simulink model "Model_8"  (R2020b)
settings: Solver=VariableStepAuto  StartTime=0.0  StopTime=10.0  RelTol=1e-3
settings Model: Creator=samar  LastModifiedBy=samar

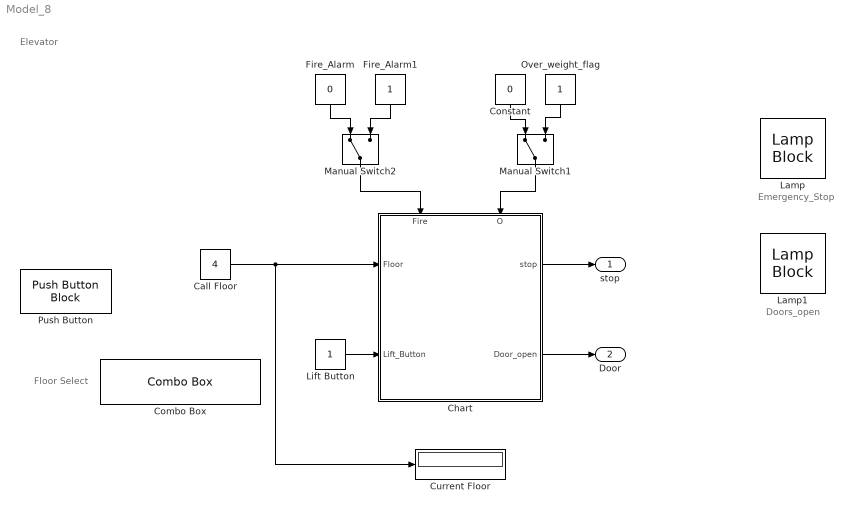
== system Model_8 ==
  note: Doors_open
  note: Emergency_Stop
  note: Floor Select
  note: Elevator
  Call Floor : Constant  Value=4
  Chart : Stateflow chart  TreatAsAtomicUnit=on
      settings: PortSchema="{\"entries\":[{\"content\":{\"sides\":[{\"content\":{\"connectorIds\":[\"In1\",\"In2\"]},\"type\":\"ConnectorPlacement.EquallySpacedRectSide\",\"uuid\":\"728db6cd-266b-43d7-bd2a-e73031a3322c\"},{\"content\":{\"connectorIds\":[\"Out1\",\"Out2\"],\"side\":\"RIGHT\"},\"type\":\"ConnectorPlacement.EquallySpacedRectSide\",\"uuid\":\"e9a7720d-fa0e-4c6c-b388-11c798bcbbca\"},{\"content\":{\"connectorIds\":[\"In3\",\"In4\"],\"side\":\"TOP\"},\"type\":\"ConnectorPlacement.EquallySpacedRectSide\",\"uuid\":\"9d412d4b-ce6a-499b-9b84-36dea582eefb\"},{\"content\":{\"connectorIds\":[],\"side\":\"HIDDEN\"},\"type\":\"ConnectorPlacement.EquallySpacedRectSide\",\"uuid\":\"5eef0b0d-4dbe-45a6-b206-45d09078b064\"}]},\"type\":\"ConnectorPlacement.EquallySpacedConnector\",\"uuid\":\"568172f0-0759-4a2b-9c34-c0fcda5b488d\"}],\"packageUris\":[\"http://schema.mathworks.com/mf0/Connector/R2020b\"],\"version\":\"1.0\"}"
  Combo Box : ComboBox  SelectedLabel=Forth_Floor
      settings: Values={{'Ground', 'First_Floor', 'Second_Floor', 'Third_Floor', 'Forth_Floor', 'Fifth_Floor'}, [0 1 2 3 4 5]}
  Constant : Constant  Value=0
  Current Floor : Display
  Fire_Alarm : Constant  Value=0
  Fire_Alarm1 : Constant
  Lamp : LampBlock
  Lamp1 : LampBlock
  Lift Button : Constant
  Manual Switch1 : ManualSwitch
  Manual Switch2 : ManualSwitch
  Over_weight_flag : Constant
  Push Button : PushButtonBlock  OnValue=0
  stop : Outport
  Door : Outport  Port=2
  wires:
  Call Floor/1 -> Chart/1(Floor), Current Floor/1
  Constant/1 -> Manual Switch1/1
  Over_weight_flag/1 -> Manual Switch1/2
  Manual Switch2/1 -> Chart/3(Fire)
  Fire_Alarm/1 -> Manual Switch2/1
  Fire_Alarm1/1 -> Manual Switch2/2
  Chart/1(stop) -> stop/1
  Lift Button/1 -> Chart/2(Lift_Button)
  Chart/2(Door_open) -> Door/1
  Manual Switch1/1 -> Chart/4(O)

== stateflow chart Model_8/Chart ==
  state Elevator
    en:
    Over_Weight(O);
    Fire_Alarm(Fire);
    state Control_Logic
      en:
      x=0;
      x = Floor;
      Over_Weight(O);
      Fire_Alarm(Fire);
      Door_open = 0;
    state Ground
      entry:
      x=6;
      Door_open = 1;
      ex:
      Door_open = 0;
    state First_Floor
      entry:
      x=6;
      Door_open = 1;
      ex:
      Door_open = 0;
    state Second_Floor
      entry:
      x=6;
      Door_open = 1;
      ex:
      Door_open = 0;
    state Third_Floor
      entry:
      x=6;
      Door_open = 1;
      ex:
      Door_open = 0;
    state Forth_Floor
      entry:
      x=6;
      Door_open = 1;
      ex:
      Door_open = 0;
    state Fifth_Floor
      entry:
      x=6;
      Door_open = 1;
      ex:
      Door_open = 0;
    Control_Logic -> Fifth_Floor [order 1] : [x == 5]
    Control_Logic -> Forth_Floor [order 2] : [x == 4]
    Control_Logic -> Third_Floor [order 3] : [x == 3]
    Control_Logic -> Second_Floor [order 4] : [x == 2]
    Control_Logic -> First_Floor [order 5] : [x == 1]
    (default) -> Control_Logic
    Control_Logic -> Ground [order 6] : [x == 0]
    First_Floor -> Control_Logic : after(6,sec)[x == 6]
    Fifth_Floor -> Control_Logic : after(6,sec)[x == 6]
    Second_Floor -> Control_Logic : after(6,sec)[x == 6]
    Third_Floor -> Control_Logic : after(6,sec)[x == 6]
    Forth_Floor -> Control_Logic : after(6,sec)[x == 6]
    Ground -> Control_Logic : after(6,sec)[x == 6]
  state Over_Weight(OW) [function]
    (default) -> (junction 64) : % Over_weight
    (junction 64) -> (junction 65) [order 1] : [OW == 1]
    (junction 64) -> (junction 66) [order 2]
    (junction 65) -> (junction 67) : {stop=1;}
    (junction 67) -> (junction 66)
    (junction 66) -> (junction 68)
  state Fire_Alarm(Fire_alarm) [function]
    (default) -> (junction 83) : % Fire_Alarm_Indicator
    (junction 83) -> (junction 84) [order 1] : [Fire_alarm == 1]
    (junction 83) -> (junction 85) [order 2]
    (junction 84) -> (junction 86) : { stop=1;}
    (junction 86) -> (junction 85)
    (junction 85) -> (junction 87)
  state Lift_Button
    en:
    Door_open = 1;
  (default) -> Elevator
  Lift_Button -> Elevator : [Lift_Button == 1]
  Elevator -> Lift_Button : [Lift_Button == 0]
  data: OW function_input; Fire_alarm function_input; Floor input; Lift_Button input; Fire input; stop output =0; Door_open output; O input; x local
